simulink model "bh_rolling_wheel_sim_simscape"  (R2022b)
settings: Solver=ode15s  StartTime=0.0  StopTime=15  RelTol=1e-6  AbsTol=1e-5  EnableMultiTasking=on
values from neighbouring files (symbols this model uses):
  X = OBJ.X_g_birth_wheel    [bh_rolling_wheel_toy_CLS.m]
  Y = OBJ.Y_g_birth_wheel    [bh_rolling_wheel_toy_CLS.m]
  Z = OBJ.Z_g_birth_wheel    [bh_rolling_wheel_toy_CLS.m]
undefined symbols (not defined in the file or in its folder): params_T
libraries: sm_lib x9, nesl_utility x7
settings Model: Creator=bhorton  LastModifiedBy=bhorton
settings SolverCC: ZeroCrossAlgorithm=Adaptive  AlgebraicLoopSolver=TrustRegion
settings DataIOCC: LimitDataPoints=on  MaxDataPoints=10000
settings OptimizationCC: LifeSpan=inf
settings DebuggingCC: UnconnectedInputMsg=warning  UnconnectedOutputMsg=warning  UnconnectedLineMsg=warning  AllowSymbolicDim=off  SFUnexpectedBacktrackingDiag=warning  SFNoUnconditionalDefaultTransitionDiag=warning  SFExecutionAtInitializationDiag=none  SFMachineParentedDataDiag=warning  ArithmeticOperatorsInVariantConditions=warning
settings ModelReferenceCC: EnableRefExpFcnMdlSchedulingChecks=on
settings SFSimCC: SimUseLocalCustomCode=off  CustomCodeUndefinedFunction=UseInterfaceOnly
settings RTWCC: RTWUseLocalCustomCode=off  DLArmComputeVersion=19.05
settings CodeAppCC: StateflowObjectComments=on
settings GRTTargetCC: TargetLangStandard=C89/C90 (ANSI)
settings ConfigComp: CovMetricSettings=dw  CovSaveCumulativeToWorkspaceVar=on  CovSaveSingleToWorkspaceVar=on  CovExternalEMLEnable=off  CovSFcnEnable=off
settings SimscapeCC: SimscapeLogType=all  SimscapeLogSimulationStatistics=on  SimscapeLogDataHistory=10000
settings ExplorerConfigSet: InternalSimMechanicsExplorerSettings="<ExplorerConfiguration><canonicalview>default</canonicalview><AnimationSetting><BasePlaybackSpeed>1.0</BasePlaybackSpeed><PlaybackSpeedFactor>1.0</PlaybackSpeedFactor></AnimationSetting><TilePanel><TileInfo><Tiles Columns=\"2\" Count=\"3\" Rows=\"2\"><Column Weight=\"0.5\"/><Column Weight=\"0.5\"/><Row Weight=\"0.4994\"/><Row Weight=\"0.5006\"/><Tile Height=\"1\" Width=\"2\" X=\"0\" Y=\"0\"/><Tile Height=\"1\" Width=\"1\" X=\"0\" Y=\"1\"/><Tile Height=\"1\" Width=\"1\" X=\"1\" Y=\"1\"/></Tiles></TileInfo><SceneInfo><SceneViewer><BGColor><R>0.60000002384185791</R><G>0.60000002384185791</G><B>0.60000002384185791</B></BGColor><Camera><DoPerspective>off</DoPerspective><Position><X>-1.55053169967245363</X><Y>-3.57091267042787441</Y><Z>1.79762407921706791</Z></Position><Center><X>0.0298580117792944799</X><Y>0.315652701739378039</Y><Z>0.371428906966243755</Z></Center><Up><X>0.188235579796397878</X><Y>0.269970042606700877</Y><Z>0.944289967432488608</Z></Up><ViewLimDist>1</ViewLimDist><YLim>2.36177470231108044</YLim><XLim>4.53695320917997602</XLim></Camera></SceneViewer><SceneViewer><BGColor><R>0.60000002384185791</R><G>0.60000002384185791</G><B>0.60000002384185791</B></BGColor><Camera><DoPerspective>off</DoPerspective><Position><X>7.9175910466799948e-08</X><Y>4.21699887787063687e-08</Y><Z>4.27096389083537709</Z></Position><Center><X>7.9175910466799948e-08</X><Y>4.21699887787063687e-08</Y><Z>0.410300941791907015</Z></Center><Up><X>0</X><Y>1</Y><Z>-0</Z></Up><ViewLimDist>1</ViewLimDist><YLim>3.25881235154394311</YLim><XLim>3.08999999999999986</XLim></Camera></SceneViewer><SceneViewer><BGColor><R>0.60000002384185791</R><G>0.60000002384185791</G><B>0.60000002384185791</B></BGColor><Camera><DoPerspective>off</DoPerspective><Position><X>2.4535844008356591</X><Y>-2.45358462381710618</Y><Z>2.45358456126027713</Z></Position><Center><X>-1.19276180646206974e-07</X><Y>-1.03705266674473913e-07</Y><Z>4.11484375746999591e-08</Z></Center><Up><X>-0.408248290463863073</X><Y>0.408248290463863073</Y><Z>0.816496580927726145</Z></Up><ViewLimDist>1</ViewLimDist><YLim>4.60865641641503565</YLim><XLim>4.36991971015930147</XLim></Camera></SceneViewer></SceneInfo></TilePanel><MechEditorPanel><Cameras/><GfxPanelCameraMap/><VideoCreator><PlaybackSpeedRatio>1.0</PlaybackSpeedRatio><FrameRate>30</FrameRate><VideoFormat>Motion JPEG AVI</VideoFormat><FrameSize>auto</FrameSize></VideoCreator></MechEditorPanel></ExplorerConfiguration>"

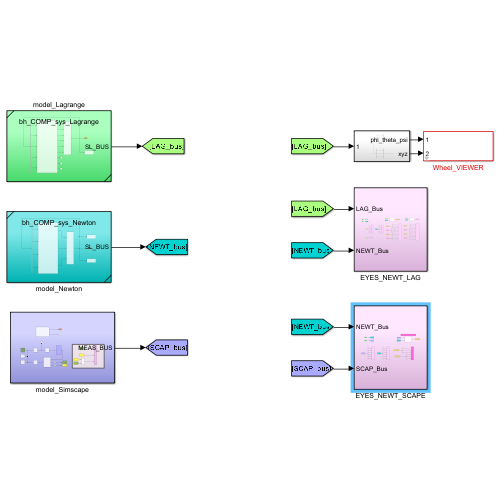
[thumbnail: Simulink's stored preview of the top-level diagram]
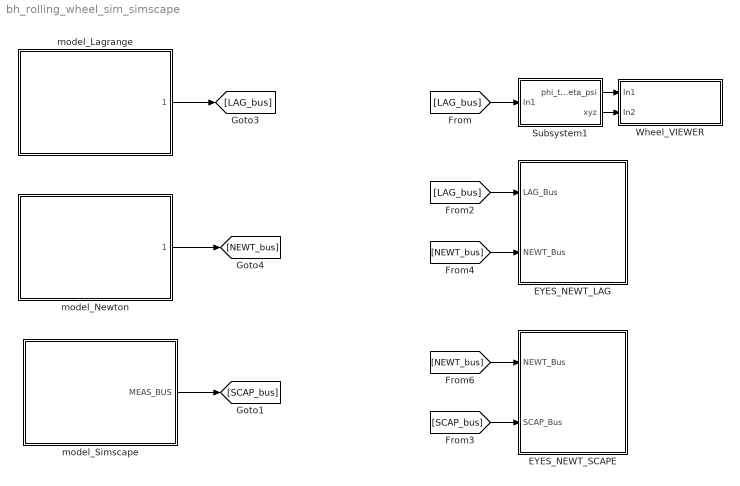
== system bh_rolling_wheel_sim_simscape ==
  EYES_NEWT_LAG : Subsystem
  EYES_NEWT_SCAPE : Subsystem
  Subsystem1 : Subsystem
  Wheel_VIEWER : Subsystem  mask{Ts=0.01, R=params_T.r, the_XLIM=[-1,1]*3, the_YLIM=[-1,1]*3, yn_create_gif=off}
      mask prompts: Ts "Sample Time"; R "Wheel radius (m)"; the_XLIM "X axis display limita"; the_YLIM "Y axis display limita"; yn_create_gif "Create a Gif animation"
      mask init:
      | tf_create_gif = false;
      | 
      | if(1 == yn_create_gif)
      |     tf_create_gif = true;
      | end
  model_Lagrange : Subsystem  ReferencedSubsystem=bh_COMP_sys_Lagrange
  model_Newton : Subsystem  ReferencedSubsystem=bh_COMP_sys_Newton
  model_Simscape : Subsystem
  wires:
  model_Lagrange/1 -> [LAG_bus]
  [LAG_bus] -> EYES_NEWT_LAG/1(LAG_Bus)
  model_Newton/1 -> [NEWT_bus]
  [NEWT_bus] -> EYES_NEWT_LAG/2(NEWT_Bus)
  [LAG_bus] -> Subsystem1/1(In1)
  Subsystem1/1(phi_theta_psi) -> Wheel_VIEWER/1(In1)
  Subsystem1/2(xyz) -> Wheel_VIEWER/2(In2)
  model_Simscape/1(MEAS_BUS) -> [SCAP_bus]
  [NEWT_bus] -> EYES_NEWT_SCAPE/1(NEWT_Bus)
  [SCAP_bus] -> EYES_NEWT_SCAPE/2(SCAP_Bus)

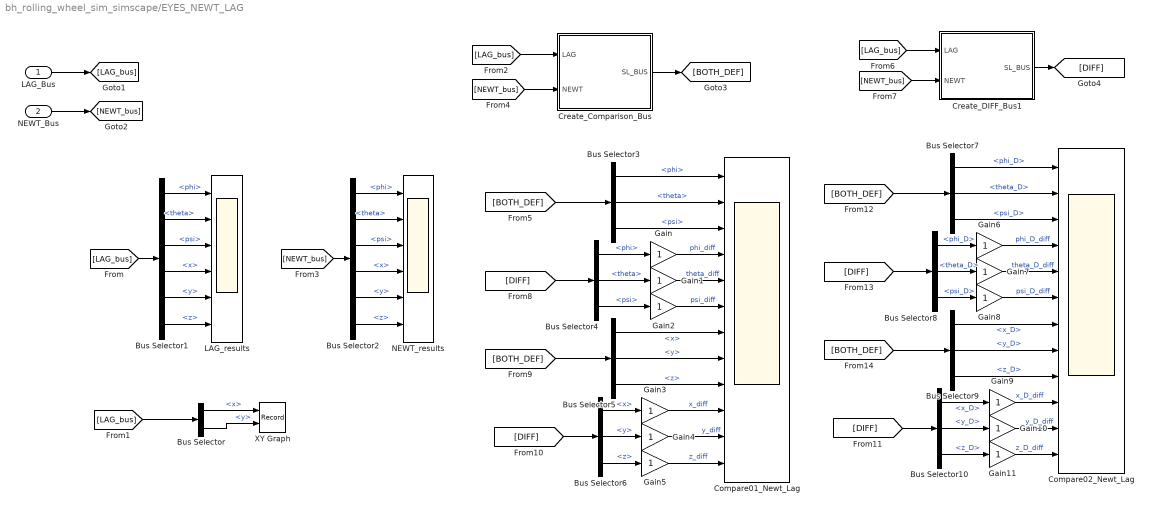
== system bh_rolling_wheel_sim_simscape/EYES_NEWT_LAG ==
  LAG_Bus : Inport
  NEWT_Bus : Inport  Port=2
  Bus Selector : BusSelector  OutputSignals=x,y
  Bus Selector1 : BusSelector  OutputSignals=phi,theta,psi,x,y,z
  Bus Selector10 : BusSelector  OutputSignals=x_D,y_D,z_D
  Bus Selector2 : BusSelector  OutputSignals=phi,theta,psi,x,y,z
  Bus Selector3 : BusSelector  OutputSignals=phi,theta,psi
  Bus Selector4 : BusSelector  OutputSignals=phi,theta,psi
  Bus Selector5 : BusSelector  OutputSignals=x,y,z
  Bus Selector6 : BusSelector  OutputSignals=x,y,z
  Bus Selector7 : BusSelector  OutputSignals=phi_D,theta_D,psi_D
  Bus Selector8 : BusSelector  OutputSignals=phi_D,theta_D,psi_D
  Bus Selector9 : BusSelector  OutputSignals=x_D,y_D,z_D
  Compare01_Newt_Lag : Scope  NumInputPorts=12
  Compare02_Newt_Lag : Scope  NumInputPorts=12
  Create_Comparison_Bus : Subsystem
  Create_DIFF_Bus1 : Subsystem
  Gain{,1..11} (12 alike) : Gain
  LAG_results : Scope  NumInputPorts=6
  NEWT_results : Scope  NumInputPorts=6
  XY Graph : Record  FileSettingsInternal="{\"entries\":[{\"content\":{\"excelSettings\":{\"content\":{},\"type\":\"Streamout.ExcelSettings\"}},\"type\":\"Streamout.FileSettingStorage\",\"uuid\":\"1ddb2a88-b2ea-40b8-bd98-e1e8a9863809\"}],\"packageUris\":[\"http://schema.mathworks.com/mf0/streamout_blocks/R2020a\"],\"version\":\"1.0\"}"  Layout=[1 1]  SignalsInternal="{\"entries\":[{\"content\":{\"signals\":[{\"content\":{\"blockPath\":[\"bh_rolling_wheel_sim_simscape/EYES_NEWT_LAG/XY Graph\"],\"channel\":[],\"dimensions\":[1],\"domain\":\"bh_rolling_wheel_sim_simscape/EYES_NEWT_LAG/XY Graph\",\"lineColor\":\"#edb120\",\"plots\":[],\"port\":1,\"sid\":[],\"signalID\":846,\"signalName\":\"<x>\"},\"type\":\"RecordBlkView.Signal\",\"uuid\":\"96332ea5-5fdc-4ca9-b00e-a419accddd88\"},{\"content\":{\"blockPath\":[\"bh_rolling_wheel_sim_simscape/EYES_NEWT_LAG/XY Graph\"],\"channel\":[],\"dimensions\":[1],\"domain\":\"bh_rolling_wheel_sim_simscape/EYES_NEWT_LAG/XY Graph\",\"lineColor\":\"#7e2f8e\",\"plots\":[],\"port\":2,\"sid\":[],\"signalID\":849,\"signalName\":\"<y>\"},\"type\":\"RecordBlkView.Signal\",\"uuid\":\"f7c696c0-69e3-4450-bb2d-fd5414803194\"}]},\"type\":\"RecordBlkView.InputSignals\",\"uuid\":\"ee3b015f-a261-4ccc-b071-21c734062a7a\"}],\"packageUris\":[\"http://schema.mathworks.com/mf0/streamout_blocks/R2020a\"],\"version\":\"1.0\"}"  VisualizationBindings="{\"xyplotplugin\":{\"info\":[{\"series\":[],\"subplotID\":1}]}}"  CompatibilityTag=XY  st=-1
  wires:
  LAG_Bus/1 -> [LAG_bus]
  [LAG_bus] -> Bus Selector1/1
  Bus Selector1/1 -> LAG_results/1  "<phi>"
  Bus Selector1/2 -> LAG_results/2  "<theta>"
  Bus Selector1/3 -> LAG_results/3  "<psi>"
  Bus Selector1/4 -> LAG_results/4  "<x>"
  Bus Selector1/5 -> LAG_results/5  "<y>"
  Bus Selector1/6 -> LAG_results/6  "<z>"
  [LAG_bus] -> Bus Selector/1
  Bus Selector/1 -> XY Graph/1  "<x>"
  Bus Selector/2 -> XY Graph/2  "<y>"
  NEWT_Bus/1 -> [NEWT_bus]
  Bus Selector2/5 -> NEWT_results/5  "<y>"
  Bus Selector2/4 -> NEWT_results/4  "<x>"
  Bus Selector2/2 -> NEWT_results/2  "<theta>"
  Bus Selector2/1 -> NEWT_results/1  "<phi>"
  Bus Selector2/6 -> NEWT_results/6  "<z>"
  [NEWT_bus] -> Bus Selector2/1
  Bus Selector2/3 -> NEWT_results/3  "<psi>"
  Create_Comparison_Bus/1(SL_BUS) -> [BOTH_DEF]
  [NEWT_bus] -> Create_Comparison_Bus/2(NEWT)
  [LAG_bus] -> Create_Comparison_Bus/1(LAG)
  [NEWT_bus] -> Create_DIFF_Bus1/2(NEWT)
  [LAG_bus] -> Create_DIFF_Bus1/1(LAG)
  Create_DIFF_Bus1/1(SL_BUS) -> [DIFF]
  [BOTH_DEF] -> Bus Selector3/1
  Bus Selector3/1 -> Compare01_Newt_Lag/1  "<phi>"
  Bus Selector3/2 -> Compare01_Newt_Lag/2  "<theta>"
  Bus Selector3/3 -> Compare01_Newt_Lag/3  "<psi>"
  Bus Selector4/1 -> Gain/1  "<phi>"
  Bus Selector4/2 -> Gain1/1  "<theta>"
  Bus Selector4/3 -> Gain2/1  "<psi>"
  [DIFF] -> Bus Selector4/1
  [BOTH_DEF] -> Bus Selector5/1
  Bus Selector5/1 -> Compare01_Newt_Lag/7  "<x>"
  Bus Selector5/2 -> Compare01_Newt_Lag/8  "<y>"
  Bus Selector5/3 -> Compare01_Newt_Lag/9  "<z>"
  Bus Selector6/2 -> Gain4/1  "<y>"
  [DIFF] -> Bus Selector6/1
  Bus Selector6/1 -> Gain3/1  "<x>"
  Bus Selector6/3 -> Gain5/1  "<z>"
  Bus Selector9/1 -> Compare02_Newt_Lag/7  "<x_D>"
  [BOTH_DEF] -> Bus Selector9/1
  Bus Selector9/3 -> Compare02_Newt_Lag/9  "<z_D>"
  Bus Selector9/2 -> Compare02_Newt_Lag/8  "<y_D>"
  Bus Selector7/1 -> Compare02_Newt_Lag/1  "<phi_D>"
  Bus Selector7/2 -> Compare02_Newt_Lag/2  "<theta_D>"
  Bus Selector7/3 -> Compare02_Newt_Lag/3  "<psi_D>"
  [DIFF] -> Bus Selector8/1
  [DIFF] -> Bus Selector10/1
  [BOTH_DEF] -> Bus Selector7/1
  Gain2/1 -> Compare01_Newt_Lag/6  "psi_diff"
  Gain/1 -> Compare01_Newt_Lag/4  "phi_diff"
  Gain1/1 -> Compare01_Newt_Lag/5  "theta_diff"
  Gain3/1 -> Compare01_Newt_Lag/10  "x_diff"
  Gain4/1 -> Compare01_Newt_Lag/11  "y_diff"
  Gain5/1 -> Compare01_Newt_Lag/12  "z_diff"
  Bus Selector8/1 -> Gain6/1  "<phi_D>"
  Bus Selector8/2 -> Gain7/1  "<theta_D>"
  Bus Selector8/3 -> Gain8/1  "<psi_D>"
  Bus Selector10/1 -> Gain9/1  "<x_D>"
  Bus Selector10/2 -> Gain10/1  "<y_D>"
  Bus Selector10/3 -> Gain11/1  "<z_D>"
  Gain6/1 -> Compare02_Newt_Lag/4  "phi_D_diff"
  Gain7/1 -> Compare02_Newt_Lag/5  "theta_D_diff"
  Gain8/1 -> Compare02_Newt_Lag/6  "psi_D_diff"
  Gain9/1 -> Compare02_Newt_Lag/10  "x_D_diff"
  Gain10/1 -> Compare02_Newt_Lag/11  "y_D_diff"
  Gain11/1 -> Compare02_Newt_Lag/12  "z_D_diff"

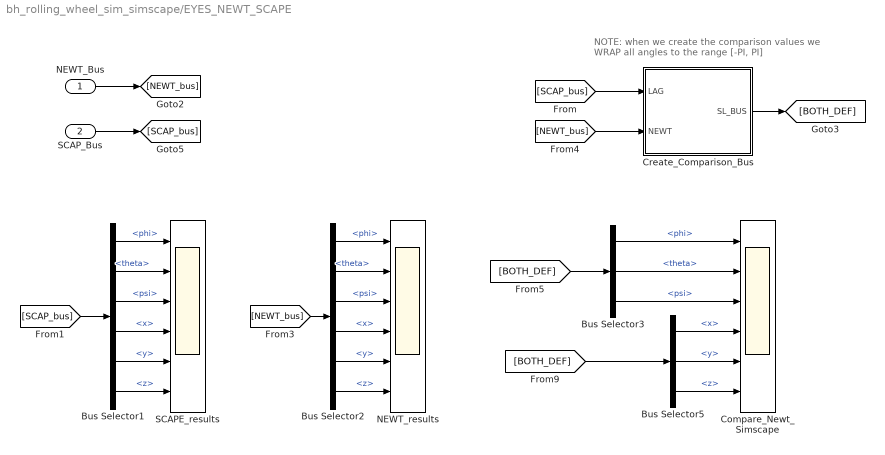
== system bh_rolling_wheel_sim_simscape/EYES_NEWT_SCAPE ==
  note: NOTE:  when we create the comparison values
      | we WRAP all angles to the range [-PI, PI]
  NEWT_Bus : Inport
  SCAP_Bus : Inport  Port=2
  Bus Selector1 : BusSelector  OutputSignals=phi,theta,psi,x,y,z
  Bus Selector2 : BusSelector  OutputSignals=phi,theta,psi,x,y,z
  Bus Selector3 : BusSelector  OutputSignals=phi,theta,psi
  Bus Selector5 : BusSelector  OutputSignals=x,y,z
  Compare_Newt_Simscape : Scope  NumInputPorts=6
  Create_Comparison_Bus : Subsystem
  NEWT_results : Scope  NumInputPorts=6
  SCAPE_results : Scope  NumInputPorts=6
  wires:
  [SCAP_bus] -> Bus Selector1/1
  Bus Selector1/1 -> SCAPE_results/1  "<phi>"
  Bus Selector1/2 -> SCAPE_results/2  "<theta>"
  Bus Selector1/3 -> SCAPE_results/3  "<psi>"
  Bus Selector1/4 -> SCAPE_results/4  "<x>"
  Bus Selector1/5 -> SCAPE_results/5  "<y>"
  Bus Selector1/6 -> SCAPE_results/6  "<z>"
  NEWT_Bus/1 -> [NEWT_bus]
  Bus Selector2/5 -> NEWT_results/5  "<y>"
  Bus Selector2/4 -> NEWT_results/4  "<x>"
  Bus Selector2/2 -> NEWT_results/2  "<theta>"
  Bus Selector2/1 -> NEWT_results/1  "<phi>"
  Bus Selector2/6 -> NEWT_results/6  "<z>"
  [NEWT_bus] -> Bus Selector2/1
  Bus Selector2/3 -> NEWT_results/3  "<psi>"
  Create_Comparison_Bus/1(SL_BUS) -> [BOTH_DEF]
  [NEWT_bus] -> Create_Comparison_Bus/2(NEWT)
  [SCAP_bus] -> Create_Comparison_Bus/1(LAG)
  [BOTH_DEF] -> Bus Selector3/1
  Bus Selector3/1 -> Compare_Newt_Simscape/1  "<phi>"
  Bus Selector3/2 -> Compare_Newt_Simscape/2  "<theta>"
  Bus Selector3/3 -> Compare_Newt_Simscape/3  "<psi>"
  [BOTH_DEF] -> Bus Selector5/1
  Bus Selector5/1 -> Compare_Newt_Simscape/4  "<x>"
  Bus Selector5/2 -> Compare_Newt_Simscape/5  "<y>"
  Bus Selector5/3 -> Compare_Newt_Simscape/6  "<z>"
  SCAP_Bus/1 -> [SCAP_bus]

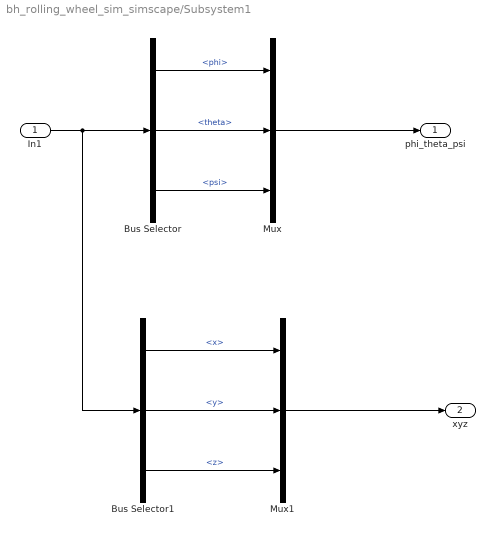
== system bh_rolling_wheel_sim_simscape/Subsystem1 ==
  In1 : Inport
  Bus Selector : BusSelector  OutputSignals=phi,theta,psi
  Bus Selector1 : BusSelector  OutputSignals=x,y,z
  Mux : Mux  Inputs=3
  Mux1 : Mux  Inputs=3
  phi_theta_psi : Outport
  xyz : Outport  Port=2
  wires:
  In1/1 -> Bus Selector1/1, Bus Selector/1
  Bus Selector/1 -> Mux/1  "<phi>"
  Bus Selector/2 -> Mux/2  "<theta>"
  Bus Selector/3 -> Mux/3  "<psi>"
  Bus Selector1/1 -> Mux1/1  "<x>"
  Bus Selector1/2 -> Mux1/2  "<y>"
  Bus Selector1/3 -> Mux1/3  "<z>"
  Mux/1 -> phi_theta_psi/1
  Mux1/1 -> xyz/1

== system bh_rolling_wheel_sim_simscape/Wheel_VIEWER ==
  In1 : Inport
  In2 : Inport  Port=2
  Level-2 MATLAB S-Function : M-S-Function  FunctionName=bh_rolling_wheel_animate_sfun  Parameters=Ts, R, the_XLIM, the_YLIM, tf_create_gif
  wires:
  In1/1 -> Level-2 MATLAB S-Function/1
  In2/1 -> Level-2 MATLAB S-Function/2

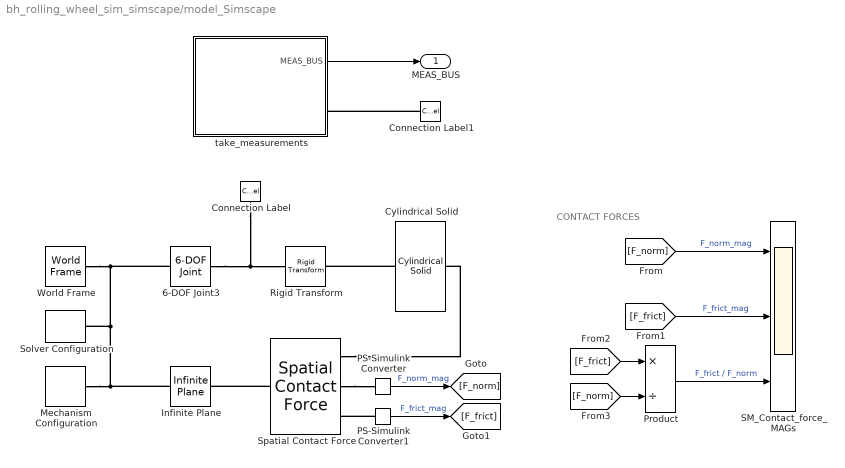
== system bh_rolling_wheel_sim_simscape/model_Simscape ==
  note: CONTACT FORCES
  6-DOF Joint3 : sm_lib/Joints/6-DOF Joint  JointMode=Normal  SenseConstraintForce=off  SenseConstraintForceX=off  SenseConstraintForceY=off  SenseConstraintForceZ=off  SenseConstraintTorque=off  SenseConstraintTorqueX=off  SenseConstraintTorqueY=off  SenseConstraintTorqueZ=off  SenseTotalForce=off  SenseTotalForceX=off  SenseTotalForceY=off  SenseTotalForceZ=off  SenseTotalTorque=off  SenseTotalTorqueX=off  SenseTotalTorqueY=off  SenseTotalTorqueZ=off  CompositeWrenchDir=FollowerOnBase  CompositeWrenchFrame=BaseFrame  PxEquilibriumPosition=0  PxEquilibriumPositionUnits=m  PxSpringStiffness=0  PxSpringStiffnessUnits=N/m  PxDampingCoefficient=0  PxDampingCoefficientUnits=N/(m/s)  PxTorqueActuationMode=NoTorque  PxMotionActuationMode=ComputedMotion  PxSensePosition=off  PxSenseVelocity=off  PxSenseAcceleration=off  PxSenseTorqueForce=off  PxSenseLowerLimitTorqueForce=off  PxSenseUpperLimitTorqueForce=off  PxLowerLimitSpecify=off  PxLowerLimitBound=-1  PxLowerLimitBoundUnits=m  PxLowerLimitStiffness=1e6  PxLowerLimitStiffnessUnits=N/m  PxLowerLimitDamping=1e3  PxLowerLimitDampingUnits=N/(m/s)  PxLowerLimitTransitionRegionWidth=1e-4  PxLowerLimitTransitionRegionWidthUnits=m  PxUpperLimitSpecify=off  PxUpperLimitBound=1  PxUpperLimitBoundUnits=m  PxUpperLimitStiffness=1e6  PxUpperLimitStiffnessUnits=N/m  PxUpperLimitDamping=1e3  PxUpperLimitDampingUnits=N/(m/s)  PxUpperLimitTransitionRegionWidth=1e-4  PxUpperLimitTransitionRegionWidthUnits=m  PxPositionTargetSpecify=on  PxPositionTargetPriority=High  PxPositionTargetValue=IC_T.x  PxPositionTargetValueUnits=m  PxVelocityTargetSpecify=on  PxVelocityTargetPriority=High  PxVelocityTargetValue=IC_T.x_dot  PxVelocityTargetValueUnits=m/s  PyEquilibriumPosition=0  PyEquilibriumPositionUnits=m  PySpringStiffness=0  PySpringStiffnessUnits=N/m  PyDampingCoefficient=0  PyDampingCoefficientUnits=N/(m/s)  PyTorqueActuationMode=NoTorque  PyMotionActuationMode=ComputedMotion  PySensePosition=off  PySenseVelocity=off  PySenseAcceleration=off  PySenseTorqueForce=off  PySenseLowerLimitTorqueForce=off  PySenseUpperLimitTorqueForce=off  PyLowerLimitSpecify=off  PyLowerLimitBound=-1  PyLowerLimitBoundUnits=m  PyLowerLimitStiffness=1e6  PyLowerLimitStiffnessUnits=N/m  PyLowerLimitDamping=1e3  PyLowerLimitDampingUnits=N/(m/s)  PyLowerLimitTransitionRegionWidth=1e-4  PyLowerLimitTransitionRegionWidthUnits=m  PyUpperLimitSpecify=off  PyUpperLimitBound=1  PyUpperLimitBoundUnits=m  PyUpperLimitStiffness=1e6  PyUpperLimitStiffnessUnits=N/m  PyUpperLimitDamping=1e3  PyUpperLimitDampingUnits=N/(m/s)  PyUpperLimitTransitionRegionWidth=1e-4  PyUpperLimitTransitionRegionWidthUnits=m  PyPositionTargetSpecify=on  PyPositionTargetPriority=High  PyPositionTargetValue=IC_T.y  PyPositionTargetValueUnits=m  PyVelocityTargetSpecify=on  PyVelocityTargetPriority=High  PyVelocityTargetValue=IC_T.y_dot  PyVelocityTargetValueUnits=m/s  PzEquilibriumPosition=0  PzEquilibriumPositionUnits=m  PzSpringStiffness=0  PzSpringStiffnessUnits=N/m  PzDampingCoefficient=0  PzDampingCoefficientUnits=N/(m/s)  PzTorqueActuationMode=NoTorque  PzMotionActuationMode=ComputedMotion  PzSensePosition=off  PzSenseVelocity=off  PzSenseAcceleration=off  PzSenseTorqueForce=off  PzSenseLowerLimitTorqueForce=off  PzSenseUpperLimitTorqueForce=off  PzLowerLimitSpecify=off  PzLowerLimitBound=-1  PzLowerLimitBoundUnits=m  PzLowerLimitStiffness=1e6  PzLowerLimitStiffnessUnits=N/m  PzLowerLimitDamping=1e3  PzLowerLimitDampingUnits=N/(m/s)  PzLowerLimitTransitionRegionWidth=1e-4  PzLowerLimitTransitionRegionWidthUnits=m  PzUpperLimitSpecify=off  PzUpperLimitBound=1  PzUpperLimitBoundUnits=m  PzUpperLimitStiffness=1e6  PzUpperLimitStiffnessUnits=N/m  PzUpperLimitDamping=1e3  PzUpperLimitDampingUnits=N/(m/s)  PzUpperLimitTransitionRegionWidth=1e-4  PzUpperLimitTransitionRegionWidthUnits=m  PzPositionTargetSpecify=on  PzPositionTargetPriority=High  PzPositionTargetValue=IC_T.z  PzPositionTargetValueUnits=m  PzVelocityTargetSpecify=on  PzVelocityTargetPriority=High  PzVelocityTargetValue=IC_T.z_dot  PzVelocityTargetValueUnits=m/s  SphEqPosRotationMethod=None  SphEqPosRotationAngleUnits=deg  SphEqPosRotationStandardAxis=+Z  SphEqPosRotationAngle=0.0  SphEqPosRotationArbitraryAxis=[0 0 1]  SphEqPosFollAlignAxisA=+X  SphEqPosBaseAlignAxisA=+Y  SphEqPosFollAlignAxisB=+Y  SphEqPosBaseAlignAxisB=+Z  SphEqPosRotationSequenceAxes=FollowerAxes  SphEqPosRotationSequence=XYX  SphEqPosRotationSequenceAngles=[0 0 0]  SphEqPosRotationSequenceAnglesUnits=deg  SphEqPosRotationMatrix=[1 0 0; 0 1 0; 0 0 1]  SphEqPosQuaternion=[1 0 0 0]  SphSpringStiffness=0  SphSpringStiffnessUnits=N*m/deg  SphDampingCoefficient=0  SphDampingCoefficientUnits=N*m/(deg/s)  SphActuateTorqueX=off  SphActuateTorqueY=off  SphActuateTorqueZ=off  SphActuateTorque=off  SphTorqueActuationMode=NoTorque  SphMotionActuationMode=ComputedMotion  SphActuationFrame=BaseFrame  SphSensePosition=off  SphSenseVelocityX=off  SphSenseVelocityY=off  SphSenseVelocityZ=off  SphSenseVelocity=off  SphSenseAccelerationX=off  SphSenseAccelerationY=off  SphSenseAccelerationZ=off  SphSenseAcceleration=off  SphSenseTorqueX=off  SphSenseTorqueY=off  SphSenseTorqueZ=off  SphSenseTorqueForce=off  SphSenseLowerLimitTorqueMag=off  SphSenseUpperLimitTorqueMag=off  SphSensingFrame=BaseFrame  SphLowerLimitSpecify=off  SphLowerLimitBound=15  SphLowerLimitBoundUnits=deg  SphLowerLimitStiffness=1e4  SphLowerLimitStiffnessUnits=N*m/deg  SphLowerLimitDamping=10  SphLowerLimitDampingUnits=N*m/(deg/s)  SphLowerLimitTransitionRegionWidth=0.1  SphLowerLimitTransitionRegionWidthUnits=deg  SphUpperLimitSpecify=off  SphUpperLimitBound=45  SphUpperLimitBoundUnits=deg  SphUpperLimitStiffness=1e4  SphUpperLimitStiffnessUnits=N*m/deg  SphUpperLimitDamping=10  SphUpperLimitDampingUnits=N*m/(deg/s)  SphUpperLimitTransitionRegionWidth=0.1  SphUpperLimitTransitionRegionWidthUnits=deg  SphPositionTargetRotationMethod=RotationSequence  SphPositionTargetRotationAngleUnits=deg  SphPositionTargetRotationStandardAxis=+Z  SphPositionTargetRotationAngle=0.0  SphPositionTargetRotationArbitraryAxis=[0 0 1]  SphPositionTargetFollAlignAxisA=+X  SphPositionTargetBaseAlignAxisA=+Y  SphPositionTargetFollAlignAxisB=+Y  SphPositionTargetBaseAlignAxisB=+Z  SphPositionTargetRotationSequenceAxes=FollowerAxes  SphPositionTargetRotationSequence=ZYX  SphPositionTargetRotationSequenceAngles=IC_T.rot_ang_ZYX  SphPositionTargetRotationSequenceAnglesUnits=rad  SphPositionTargetRotationMatrix=[1 0 0; 0 1 0; 0 0 1]  SphPositionTargetQuaternion=[1 0 0 0]  SphPositionTargetSpecify=on  SphPositionTargetPriority=High  SphVelocityTargetValue=IC_T.rot_vel_ZYX  SphVelocityTargetValueUnits=rad/s  SphVelocityTargetSpecify=on  SphVelocityTargetPriority=High  SphVelocityTargetInFollowerFrame=on
  Connection Label : ConnectionLabel  Label=CoM
  Connection Label1 : ConnectionLabel  Label=CoM
  Cylindrical Solid : sm_lib/Body Elements/Cylindrical Solid  GraphicAmbientColor=[0.15 0.15 0.15 1.0]  BasedOnType=Mass  CenterOfMass=[0 0 0]  CenterOfMassUnits=m  GraphicDiffuseColor=[0.6 0.6 1.0]  CylinderLength=params_T.r/100  CylinderLengthUnits=m  CylinderRadius=params_T.r  CylinderRadiusUnits=m  Density=1000  DensityUnits=kg/m^3  DoExposeReferenceFrame=on  GraphicEmissiveColor=[0.0 0.0 0.0 1.0]  ExportEntireGeometry=on  SerializedFrames=<Frames/>  MarkerShape=Sphere  MarkerSize=10  GraphicType=FromGeometry  InertiaType=Custom  Mass=params_T.m  MassUnits=kg  MomentsOfInertia=params.I_mome_for_simscape  MomentsOfInertiaUnits=kg*m^2  GraphicOpacity=1.0  ProductsOfInertia=params.I_prod_for_simscape  ProductsOfInertiaUnits=kg*m^2  GraphicShininess=75  GraphicSpecularColor=[0.5 0.5 0.5 1.0]  GraphicVisPropType=SimpleVisualProperties
  Infinite Plane : sm_lib/Curves and Surfaces/Infinite Plane  GraphicType=Rectangle  GraphicPlaneWidth=6  GraphicPlaneWidthUnits=m  GraphicPlaneHeight=6  GraphicPlaneHeightUnits=m  GraphicVisPropType=SimpleVisualProperties  GraphicDiffuseColor=[0.5 0.5 0.5]  GraphicOpacity=0.25  GraphicSpecularColor=[0.5 0.5 0.5 1.0]  GraphicAmbientColor=[0.15 0.15 0.15 1.0]  GraphicEmissiveColor=[0.0 0.0 0.0 1.0]  GraphicShininess=75
  Mechanism Configuration : sm_lib/Utilities/Mechanism Configuration  UniformGravity=Constant  GravityVector=[0 0 -9.80665]  GravityUnits=m/s^2  LinearizationDelta=0.001  JointModeTransitionNonlinearIterations=2
  PS-Simulink Converter : nesl_utility/PS-Simulink Converter  PhysicalDomain=network_engine_domain  SubClassName=ps_output  LeftPortType=input  RightPortType=output  PseudoPeriodic=off  Frequencies=[]  VectorFormat=1-D array  Unit=N  AffineConversion=off
  PS-Simulink Converter1 : nesl_utility/PS-Simulink Converter  PhysicalDomain=network_engine_domain  SubClassName=ps_output  LeftPortType=input  RightPortType=output  PseudoPeriodic=off  Frequencies=[]  VectorFormat=1-D array  Unit=N  AffineConversion=off
  Product : Product  Inputs=*/
  Rigid Transform : sm_lib/Frames and Transforms/Rigid Transform  TranslationMethod=None  TranslationStandardOffset=0  TranslationLengthUnit=m  TranslationStandardAxis=+Z  TranslationCartesianOffset=[0 0 0]  TranslationROffset=0  TranslationROffsetUnits=m  TranslationZOffset=0  TranslationZOffsetUnits=m  TranslationThetaOffset=0  TranslationThetaOffsetUnits=deg  RotationMethod=AlignedAxes  RotationAngleUnits=deg  RotationStandardAxis=+Z  RotationAngle=0.0  RotationArbitraryAxis=[0 0 1]  FollAlignAxisA=+Y  BaseAlignAxisA=+Z  FollAlignAxisB=+X  BaseAlignAxisB=+Y  RotationSequenceAxes=FollowerAxes  RotationSequence=XYX  RotationSequenceAngles=[0 0 0]  RotationSequenceAnglesUnits=deg  RotationMatrix=[1 0 0; 0 1 0; 0 0 1]  Quaternion=[1 0 0 0]
  SM_Contact_force_MAGs : Scope  NumInputPorts=3
  Solver Configuration : nesl_utility/Solver Configuration  PhysicalDomain=network_engine_domain  SubClassName=solver  LeftPortType=input  RightPortType=generic  Tones=[]  Harmonics=[]  SimulateNoise=off  Profile=off  UseLocalSampling=off  EnableSwitchedLinearOptims=on  FrequencyDomain=off  UseCCode=off  RelTol=0.001  AbsTol=1e-06  MinStep=1e-09  ToWorkspace=off  RevertToSquareIcSolve=off  NumHomotopyIterations=100  PhasorMode=off  PhasorModeNumHarmonics=1  ConsistencySolver=NEWTON_FTOL  IndexReductionMethod=DerivativeReplacement  DoDC=off  ResidualTolerance=1e-09  ConsistencyTolSource=GLOBAL  ConsistencyAbsTol=0.001  ConsistencyRelTol=0.001  ConsistencyTolFactor=0.001  UseLocalSolver=off  LocalSolverChoice=NE_BACKWARD_EULER_ADVANCER  ResolveIndetEquations=on  FunctionEvalNumThread=1  LocalSolverSampleTime=0.001  DoFixedCost=off  MaxNonlinIter=3  MaxModeIter=2  ComputeImpulses=off  ImpulseIterations=2  LinearAlgebra=Sparse  LinearAlgebraNumThread=0  EquationFormulation=NE_TIME_EF  DelaysMemoryBudget=1024  AutomaticFiltering=on  FilteringTimeConstant=0.001  PartitionStorageMethod=AS_NEEDED  PartitionMemoryBudget=1024  PartitionMethod=FAST
  Spatial Contact Force : sm_lib/Forces and Torques/Spatial Contact Force  SenseContactBaseRotation=off  SenseContactBaseTranslation=off  CoefficientOfDynamicFriction=contact.Ff_codyn  CoefficientOfStaticFriction=contact.Ff_costat  NormalDamping=contact.Nf_damp  NormalDampingUnits=N/(m/s)  SenseContactSignal=off  NormalStiffness=contact.Nf_stiff  NormalStiffnessUnits=N/m  FrictionalCriticalVelocity=contact.Ff_critvel  FrictionalCriticalVelocityUnits=m/s  ZeroCrossDetectContactStartAndEnd=off  SenseContactFollowerRotation=off  SenseContactFollowerTranslation=off  FrictionType=SmoothStickSlip  SenseFrictionalForceMagnitude=on  SenseNormalForceMagnitude=on  NormalForceType=SmoothSpringDamper  SenseNormalVelocity=off  SenseSeparationDistance=off  SenseTangentialVelocity=off  NormalTransitionRegionWidth=contact.Nf_trwidth  NormalTransitionRegionWidthUnits=m
  World Frame : sm_lib/Frames and Transforms/World Frame
  take_measurements : Subsystem
  MEAS_BUS : Outport
  wires:
  take_measurements/1(MEAS_BUS) -> MEAS_BUS/1
  PS-Simulink Converter/1 -> [F_norm]  "F_norm_mag"
  PS-Simulink Converter1/1 -> [F_frict]  "F_frict_mag"
  Product/1 -> SM_Contact_force_MAGs/3  "F_frict / F_norm"
  [F_frict] -> SM_Contact_force_MAGs/2  "F_frict_mag"
  [F_norm] -> SM_Contact_force_MAGs/1  "F_norm_mag"
  [F_norm] -> Product/2
  [F_frict] -> Product/1
  connections:
  Mechanism Configuration/RConn1 -- Infinite Plane/LConn1 -- World Frame/RConn1 -- 6-DOF Joint3/LConn1 -- Solver Configuration/RConn1
  6-DOF Joint3/RConn1 -- Connection Label/LConn1 -- Rigid Transform/LConn1
  Cylindrical Solid/RConn1 -- Rigid Transform/RConn1
  Spatial Contact Force/LConn1 -- Infinite Plane/RConn1
  Spatial Contact Force/RConn1 -- Cylindrical Solid/LConn1
  Connection Label1/LConn1 -- take_measurements/RConn1
  Spatial Contact Force/RConn2 -- PS-Simulink Converter/LConn1
  PS-Simulink Converter1/LConn1 -- Spatial Contact Force/RConn3

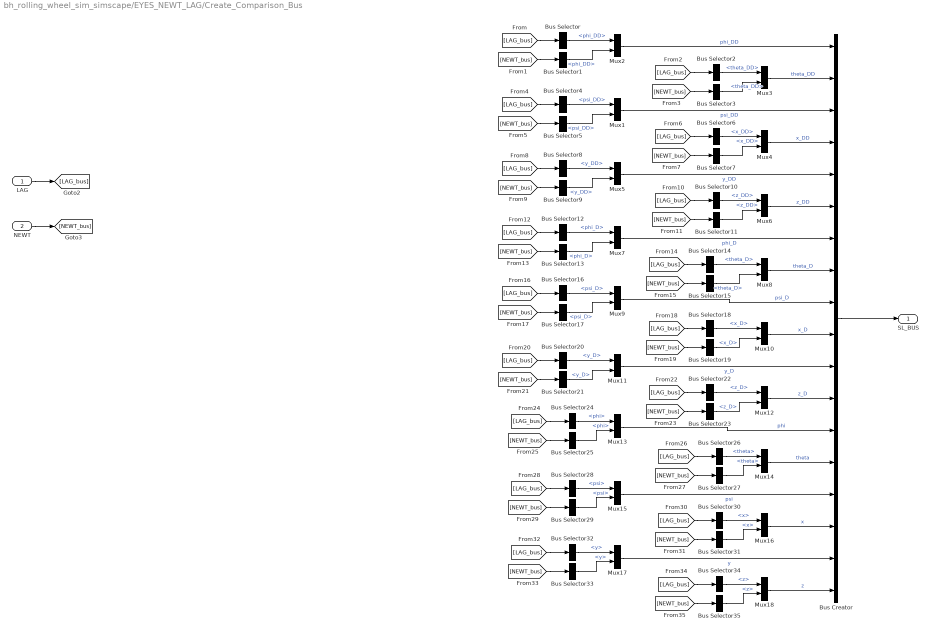
== system bh_rolling_wheel_sim_simscape/EYES_NEWT_LAG/Create_Comparison_Bus ==
  LAG : Inport
  NEWT : Inport  Port=2
  Bus Creator : BusCreator  Inputs=18
  Bus Selector : BusSelector  OutputSignals=phi_DD
  Bus Selector1 : BusSelector  OutputSignals=phi_DD
  Bus Selector10 : BusSelector  OutputSignals=z_DD
  Bus Selector11 : BusSelector  OutputSignals=z_DD
  Bus Selector12 : BusSelector  OutputSignals=phi_D
  Bus Selector13 : BusSelector  OutputSignals=phi_D
  Bus Selector14 : BusSelector  OutputSignals=theta_D
  Bus Selector15 : BusSelector  OutputSignals=theta_D
  Bus Selector16 : BusSelector  OutputSignals=psi_D
  Bus Selector17 : BusSelector  OutputSignals=psi_D
  Bus Selector18 : BusSelector  OutputSignals=x_D
  Bus Selector19 : BusSelector  OutputSignals=x_D
  Bus Selector2 : BusSelector  OutputSignals=theta_DD
  Bus Selector20 : BusSelector  OutputSignals=y_D
  Bus Selector21 : BusSelector  OutputSignals=y_D
  Bus Selector22 : BusSelector  OutputSignals=z_D
  Bus Selector23 : BusSelector  OutputSignals=z_D
  Bus Selector24 : BusSelector  OutputSignals=phi
  Bus Selector25 : BusSelector  OutputSignals=phi
  Bus Selector26 : BusSelector  OutputSignals=theta
  Bus Selector27 : BusSelector  OutputSignals=theta
  Bus Selector28 : BusSelector  OutputSignals=psi
  Bus Selector29 : BusSelector  OutputSignals=psi
  Bus Selector3 : BusSelector  OutputSignals=theta_DD
  Bus Selector30 : BusSelector  OutputSignals=x
  Bus Selector31 : BusSelector  OutputSignals=x
  Bus Selector32 : BusSelector  OutputSignals=y
  Bus Selector33 : BusSelector  OutputSignals=y
  Bus Selector34 : BusSelector  OutputSignals=z
  Bus Selector35 : BusSelector  OutputSignals=z
  Bus Selector4 : BusSelector  OutputSignals=psi_DD
  Bus Selector5 : BusSelector  OutputSignals=psi_DD
  Bus Selector6 : BusSelector  OutputSignals=x_DD
  Bus Selector7 : BusSelector  OutputSignals=x_DD
  Bus Selector8 : BusSelector  OutputSignals=y_DD
  Bus Selector9 : BusSelector  OutputSignals=y_DD
  Mux{1..18} (18 alike) : Mux  Inputs=2
  SL_BUS : Outport
  wires:
  NEWT/1 -> [NEWT_bus]
  LAG/1 -> [LAG_bus]
  [LAG_bus] -> Bus Selector/1
  [NEWT_bus] -> Bus Selector1/1
  Bus Selector/1 -> Mux2/1  "<phi_DD>"
  Bus Selector1/1 -> Mux2/2  "<phi_DD>"
  Mux3/1 -> Bus Creator/2  "theta_DD"
  Mux13/1 -> Bus Creator/13  "phi"
  Mux18/1 -> Bus Creator/18  "z"
  Mux16/1 -> Bus Creator/16  "x"
  Mux15/1 -> Bus Creator/15  "psi"
  Mux9/1 -> Bus Creator/9  "psi_D"
  Mux8/1 -> Bus Creator/8  "theta_D"
  Mux12/1 -> Bus Creator/12  "z_D"
  Mux11/1 -> Bus Creator/11  "y_D"
  Mux17/1 -> Bus Creator/17  "y"
  Mux5/1 -> Bus Creator/5  "y_DD"
  Mux14/1 -> Bus Creator/14  "theta"
  Bus Creator/1 -> SL_BUS/1
  Mux7/1 -> Bus Creator/7  "phi_D"
  Mux10/1 -> Bus Creator/10  "x_D"
  Mux6/1 -> Bus Creator/6  "z_DD"
  Mux4/1 -> Bus Creator/4  "x_DD"
  Mux1/1 -> Bus Creator/3  "psi_DD"
  Mux2/1 -> Bus Creator/1  "phi_DD"
  [LAG_bus] -> Bus Selector2/1
  [NEWT_bus] -> Bus Selector3/1
  Bus Selector2/1 -> Mux3/1  "<theta_DD>"
  Bus Selector3/1 -> Mux3/2  "<theta_DD>"
  Bus Selector5/1 -> Mux1/2  "<psi_DD>"
  [LAG_bus] -> Bus Selector4/1
  Bus Selector4/1 -> Mux1/1  "<psi_DD>"
  [NEWT_bus] -> Bus Selector5/1
  Bus Selector6/1 -> Mux4/1  "<x_DD>"
  [NEWT_bus] -> Bus Selector7/1
  [LAG_bus] -> Bus Selector6/1
  Bus Selector7/1 -> Mux4/2  "<x_DD>"
  Bus Selector8/1 -> Mux5/1  "<y_DD>"
  [LAG_bus] -> Bus Selector8/1
  [NEWT_bus] -> Bus Selector9/1
  Bus Selector9/1 -> Mux5/2  "<y_DD>"
  Bus Selector10/1 -> Mux6/1  "<z_DD>"
  Bus Selector11/1 -> Mux6/2  "<z_DD>"
  [LAG_bus] -> Bus Selector10/1
  [NEWT_bus] -> Bus Selector11/1
  Bus Selector13/1 -> Mux7/2  "<phi_D>"
  [LAG_bus] -> Bus Selector12/1
  Bus Selector12/1 -> Mux7/1  "<phi_D>"
  [NEWT_bus] -> Bus Selector13/1
  Bus Selector14/1 -> Mux8/1  "<theta_D>"
  [NEWT_bus] -> Bus Selector15/1
  [LAG_bus] -> Bus Selector14/1
  Bus Selector15/1 -> Mux8/2  "<theta_D>"
  [NEWT_bus] -> Bus Selector17/1
  [LAG_bus] -> Bus Selector16/1
  Bus Selector17/1 -> Mux9/2  "<psi_D>"
  Bus Selector16/1 -> Mux9/1  "<psi_D>"
  Bus Selector19/1 -> Mux10/2  "<x_D>"
  [LAG_bus] -> Bus Selector18/1
  Bus Selector18/1 -> Mux10/1  "<x_D>"
  [NEWT_bus] -> Bus Selector19/1
  Bus Selector20/1 -> Mux11/1  "<y_D>"
  [LAG_bus] -> Bus Selector20/1
  [NEWT_bus] -> Bus Selector21/1
  Bus Selector21/1 -> Mux11/2  "<y_D>"
  [NEWT_bus] -> Bus Selector23/1
  Bus Selector23/1 -> Mux12/2  "<z_D>"
  [LAG_bus] -> Bus Selector22/1
  Bus Selector22/1 -> Mux12/1  "<z_D>"
  [NEWT_bus] -> Bus Selector25/1
  [LAG_bus] -> Bus Selector24/1
  Bus Selector24/1 -> Mux13/1  "<phi>"
  Bus Selector25/1 -> Mux13/2  "<phi>"
  [LAG_bus] -> Bus Selector26/1
  [NEWT_bus] -> Bus Selector27/1
  Bus Selector27/1 -> Mux14/2  "<theta>"
  Bus Selector26/1 -> Mux14/1  "<theta>"
  Bus Selector29/1 -> Mux15/2  "<psi>"
  Bus Selector28/1 -> Mux15/1  "<psi>"
  [LAG_bus] -> Bus Selector28/1
  [NEWT_bus] -> Bus Selector29/1
  Bus Selector31/1 -> Mux16/2  "<x>"
  Bus Selector30/1 -> Mux16/1  "<x>"
  [LAG_bus] -> Bus Selector30/1
  [NEWT_bus] -> Bus Selector31/1
  [NEWT_bus] -> Bus Selector33/1
  [LAG_bus] -> Bus Selector32/1
  Bus Selector32/1 -> Mux17/1  "<y>"
  Bus Selector33/1 -> Mux17/2  "<y>"
  [NEWT_bus] -> Bus Selector35/1
  Bus Selector35/1 -> Mux18/2  "<z>"
  [LAG_bus] -> Bus Selector34/1
  Bus Selector34/1 -> Mux18/1  "<z>"

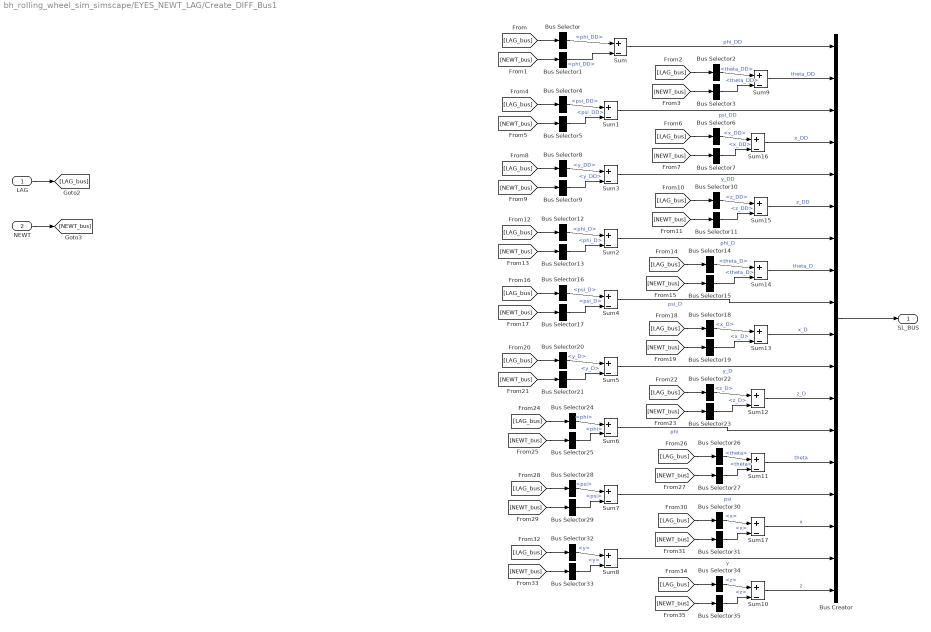
== system bh_rolling_wheel_sim_simscape/EYES_NEWT_LAG/Create_DIFF_Bus1 ==
  LAG : Inport
  NEWT : Inport  Port=2
  Bus Creator : BusCreator  Inputs=18
  Bus Selector : BusSelector  OutputSignals=phi_DD
  Bus Selector1 : BusSelector  OutputSignals=phi_DD
  Bus Selector10 : BusSelector  OutputSignals=z_DD
  Bus Selector11 : BusSelector  OutputSignals=z_DD
  Bus Selector12 : BusSelector  OutputSignals=phi_D
  Bus Selector13 : BusSelector  OutputSignals=phi_D
  Bus Selector14 : BusSelector  OutputSignals=theta_D
  Bus Selector15 : BusSelector  OutputSignals=theta_D
  Bus Selector16 : BusSelector  OutputSignals=psi_D
  Bus Selector17 : BusSelector  OutputSignals=psi_D
  Bus Selector18 : BusSelector  OutputSignals=x_D
  Bus Selector19 : BusSelector  OutputSignals=x_D
  Bus Selector2 : BusSelector  OutputSignals=theta_DD
  Bus Selector20 : BusSelector  OutputSignals=y_D
  Bus Selector21 : BusSelector  OutputSignals=y_D
  Bus Selector22 : BusSelector  OutputSignals=z_D
  Bus Selector23 : BusSelector  OutputSignals=z_D
  Bus Selector24 : BusSelector  OutputSignals=phi
  Bus Selector25 : BusSelector  OutputSignals=phi
  Bus Selector26 : BusSelector  OutputSignals=theta
  Bus Selector27 : BusSelector  OutputSignals=theta
  Bus Selector28 : BusSelector  OutputSignals=psi
  Bus Selector29 : BusSelector  OutputSignals=psi
  Bus Selector3 : BusSelector  OutputSignals=theta_DD
  Bus Selector30 : BusSelector  OutputSignals=x
  Bus Selector31 : BusSelector  OutputSignals=x
  Bus Selector32 : BusSelector  OutputSignals=y
  Bus Selector33 : BusSelector  OutputSignals=y
  Bus Selector34 : BusSelector  OutputSignals=z
  Bus Selector35 : BusSelector  OutputSignals=z
  Bus Selector4 : BusSelector  OutputSignals=psi_DD
  Bus Selector5 : BusSelector  OutputSignals=psi_DD
  Bus Selector6 : BusSelector  OutputSignals=x_DD
  Bus Selector7 : BusSelector  OutputSignals=x_DD
  Bus Selector8 : BusSelector  OutputSignals=y_DD
  Bus Selector9 : BusSelector  OutputSignals=y_DD
  Sum{,1..17} (18 alike) : Sum  Inputs=+|-
  SL_BUS : Outport
  wires:
  NEWT/1 -> [NEWT_bus]
  LAG/1 -> [LAG_bus]
  [LAG_bus] -> Bus Selector/1
  [NEWT_bus] -> Bus Selector1/1
  Bus Selector/1 -> Sum/1  "<phi_DD>"
  Bus Selector1/1 -> Sum/2  "<phi_DD>"
  Sum9/1 -> Bus Creator/2  "theta_DD"
  Sum6/1 -> Bus Creator/13  "phi"
  Sum10/1 -> Bus Creator/18  "z"
  Sum17/1 -> Bus Creator/16  "x"
  Sum7/1 -> Bus Creator/15  "psi"
  Sum4/1 -> Bus Creator/9  "psi_D"
  Sum14/1 -> Bus Creator/8  "theta_D"
  Sum12/1 -> Bus Creator/12  "z_D"
  Sum5/1 -> Bus Creator/11  "y_D"
  Sum8/1 -> Bus Creator/17  "y"
  Sum3/1 -> Bus Creator/5  "y_DD"
  Sum11/1 -> Bus Creator/14  "theta"
  Bus Creator/1 -> SL_BUS/1
  Sum2/1 -> Bus Creator/7  "phi_D"
  Sum13/1 -> Bus Creator/10  "x_D"
  Sum15/1 -> Bus Creator/6  "z_DD"
  Sum16/1 -> Bus Creator/4  "x_DD"
  Sum1/1 -> Bus Creator/3  "psi_DD"
  Sum/1 -> Bus Creator/1  "phi_DD"
  [LAG_bus] -> Bus Selector2/1
  [NEWT_bus] -> Bus Selector3/1
  Bus Selector2/1 -> Sum9/1  "<theta_DD>"
  Bus Selector3/1 -> Sum9/2  "<theta_DD>"
  [LAG_bus] -> Bus Selector4/1
  [NEWT_bus] -> Bus Selector5/1
  [NEWT_bus] -> Bus Selector7/1
  [LAG_bus] -> Bus Selector6/1
  [LAG_bus] -> Bus Selector8/1
  [NEWT_bus] -> Bus Selector9/1
  [LAG_bus] -> Bus Selector10/1
  [NEWT_bus] -> Bus Selector11/1
  [LAG_bus] -> Bus Selector12/1
  [NEWT_bus] -> Bus Selector13/1
  [NEWT_bus] -> Bus Selector15/1
  [LAG_bus] -> Bus Selector14/1
  [NEWT_bus] -> Bus Selector17/1
  [LAG_bus] -> Bus Selector16/1
  [LAG_bus] -> Bus Selector18/1
  [NEWT_bus] -> Bus Selector19/1
  [LAG_bus] -> Bus Selector20/1
  [NEWT_bus] -> Bus Selector21/1
  [NEWT_bus] -> Bus Selector23/1
  [LAG_bus] -> Bus Selector22/1
  [NEWT_bus] -> Bus Selector25/1
  [LAG_bus] -> Bus Selector24/1
  [LAG_bus] -> Bus Selector26/1
  [NEWT_bus] -> Bus Selector27/1
  [LAG_bus] -> Bus Selector28/1
  [NEWT_bus] -> Bus Selector29/1
  [LAG_bus] -> Bus Selector30/1
  [NEWT_bus] -> Bus Selector31/1
  [NEWT_bus] -> Bus Selector33/1
  [LAG_bus] -> Bus Selector32/1
  [NEWT_bus] -> Bus Selector35/1
  [LAG_bus] -> Bus Selector34/1
  Bus Selector4/1 -> Sum1/1  "<psi_DD>"
  Bus Selector5/1 -> Sum1/2  "<psi_DD>"
  Bus Selector8/1 -> Sum3/1  "<y_DD>"
  Bus Selector9/1 -> Sum3/2  "<y_DD>"
  Bus Selector12/1 -> Sum2/1  "<phi_D>"
  Bus Selector13/1 -> Sum2/2  "<phi_D>"
  Bus Selector16/1 -> Sum4/1  "<psi_D>"
  Bus Selector17/1 -> Sum4/2  "<psi_D>"
  Bus Selector20/1 -> Sum5/1  "<y_D>"
  Bus Selector21/1 -> Sum5/2  "<y_D>"
  Bus Selector24/1 -> Sum6/1  "<phi>"
  Bus Selector25/1 -> Sum6/2  "<phi>"
  Bus Selector28/1 -> Sum7/1  "<psi>"
  Bus Selector29/1 -> Sum7/2  "<psi>"
  Bus Selector32/1 -> Sum8/1  "<y>"
  Bus Selector33/1 -> Sum8/2  "<y>"
  Bus Selector6/1 -> Sum16/1  "<x_DD>"
  Bus Selector7/1 -> Sum16/2  "<x_DD>"
  Bus Selector10/1 -> Sum15/1  "<z_DD>"
  Bus Selector11/1 -> Sum15/2  "<z_DD>"
  Bus Selector14/1 -> Sum14/1  "<theta_D>"
  Bus Selector15/1 -> Sum14/2  "<theta_D>"
  Bus Selector18/1 -> Sum13/1  "<x_D>"
  Bus Selector19/1 -> Sum13/2  "<x_D>"
  Bus Selector22/1 -> Sum12/1  "<z_D>"
  Bus Selector23/1 -> Sum12/2  "<z_D>"
  Bus Selector26/1 -> Sum11/1  "<theta>"
  Bus Selector27/1 -> Sum11/2  "<theta>"
  Bus Selector30/1 -> Sum17/1  "<x>"
  Bus Selector31/1 -> Sum17/2  "<x>"
  Bus Selector34/1 -> Sum10/1  "<z>"
  Bus Selector35/1 -> Sum10/2  "<z>"

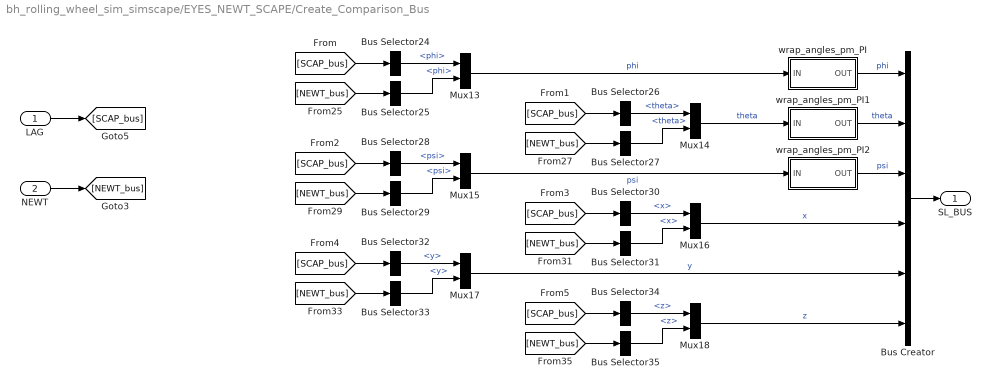
== system bh_rolling_wheel_sim_simscape/EYES_NEWT_SCAPE/Create_Comparison_Bus ==
  LAG : Inport
  NEWT : Inport  Port=2
  Bus Creator : BusCreator  Inputs=6
  Bus Selector24 : BusSelector  OutputSignals=phi
  Bus Selector25 : BusSelector  OutputSignals=phi
  Bus Selector26 : BusSelector  OutputSignals=theta
  Bus Selector27 : BusSelector  OutputSignals=theta
  Bus Selector28 : BusSelector  OutputSignals=psi
  Bus Selector29 : BusSelector  OutputSignals=psi
  Bus Selector30 : BusSelector  OutputSignals=x
  Bus Selector31 : BusSelector  OutputSignals=x
  Bus Selector32 : BusSelector  OutputSignals=y
  Bus Selector33 : BusSelector  OutputSignals=y
  Bus Selector34 : BusSelector  OutputSignals=z
  Bus Selector35 : BusSelector  OutputSignals=z
  Mux{13..18} (6 alike) : Mux  Inputs=2
  wrap_angles_pm_PI : Subsystem
  wrap_angles_pm_PI1 : Subsystem
  wrap_angles_pm_PI2 : Subsystem
  SL_BUS : Outport
  wires:
  NEWT/1 -> [NEWT_bus]
  LAG/1 -> [SCAP_bus]
  wrap_angles_pm_PI/1(OUT) -> Bus Creator/1  "phi"
  Mux18/1 -> Bus Creator/6  "z"
  Mux16/1 -> Bus Creator/4  "x"
  wrap_angles_pm_PI2/1(OUT) -> Bus Creator/3  "psi"
  Mux17/1 -> Bus Creator/5  "y"
  wrap_angles_pm_PI1/1(OUT) -> Bus Creator/2  "theta"
  Bus Creator/1 -> SL_BUS/1
  [NEWT_bus] -> Bus Selector25/1
  [SCAP_bus] -> Bus Selector24/1
  Bus Selector24/1 -> Mux13/1  "<phi>"
  Bus Selector25/1 -> Mux13/2  "<phi>"
  [SCAP_bus] -> Bus Selector26/1
  [NEWT_bus] -> Bus Selector27/1
  Bus Selector27/1 -> Mux14/2  "<theta>"
  Bus Selector26/1 -> Mux14/1  "<theta>"
  Bus Selector29/1 -> Mux15/2  "<psi>"
  Bus Selector28/1 -> Mux15/1  "<psi>"
  [SCAP_bus] -> Bus Selector28/1
  [NEWT_bus] -> Bus Selector29/1
  Bus Selector31/1 -> Mux16/2  "<x>"
  Bus Selector30/1 -> Mux16/1  "<x>"
  [SCAP_bus] -> Bus Selector30/1
  [NEWT_bus] -> Bus Selector31/1
  [NEWT_bus] -> Bus Selector33/1
  [SCAP_bus] -> Bus Selector32/1
  Bus Selector32/1 -> Mux17/1  "<y>"
  Bus Selector33/1 -> Mux17/2  "<y>"
  [NEWT_bus] -> Bus Selector35/1
  Bus Selector35/1 -> Mux18/2  "<z>"
  [SCAP_bus] -> Bus Selector34/1
  Bus Selector34/1 -> Mux18/1  "<z>"
  Mux15/1 -> wrap_angles_pm_PI2/1(IN)  "psi"
  Mux14/1 -> wrap_angles_pm_PI1/1(IN)  "theta"
  Mux13/1 -> wrap_angles_pm_PI/1(IN)  "phi"

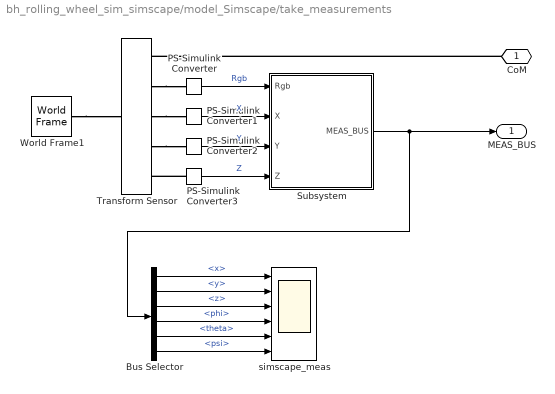
== system bh_rolling_wheel_sim_simscape/model_Simscape/take_measurements ==
  Bus Selector : BusSelector  OutputSignals=x,y,z,phi,theta,psi
  PS-Simulink Converter : nesl_utility/PS-Simulink Converter  PhysicalDomain=network_engine_domain  SubClassName=ps_output  LeftPortType=input  RightPortType=output  PseudoPeriodic=off  Frequencies=[]  VectorFormat=1-D array  Unit=m  AffineConversion=off
  PS-Simulink Converter1 : nesl_utility/PS-Simulink Converter  PhysicalDomain=network_engine_domain  SubClassName=ps_output  LeftPortType=input  RightPortType=output  PseudoPeriodic=off  Frequencies=[]  VectorFormat=1-D array  Unit=m  AffineConversion=off
  PS-Simulink Converter2 : nesl_utility/PS-Simulink Converter  PhysicalDomain=network_engine_domain  SubClassName=ps_output  LeftPortType=input  RightPortType=output  PseudoPeriodic=off  Frequencies=[]  VectorFormat=1-D array  Unit=m  AffineConversion=off
  PS-Simulink Converter3 : nesl_utility/PS-Simulink Converter  PhysicalDomain=network_engine_domain  SubClassName=ps_output  LeftPortType=input  RightPortType=output  PseudoPeriodic=off  Frequencies=[]  VectorFormat=1-D array  Unit=1  AffineConversion=off
  Subsystem : Subsystem
  Transform Sensor : sm_lib/Frames and Transforms/Transform Sensor  MeasurementFrame=World  SenseAngle=off  SenseAxis=off  SenseQ=off  SenseR=on  SenseRotationSequence=off  RotationSequence=XYX  SenseOmegaX=off  SenseOmegaY=off  SenseOmegaZ=off  SenseQDot=off  SenseRDot=off  SenseAlphaX=off  SenseAlphaY=off  SenseAlphaZ=off  SenseQDDot=off  SenseRDDot=off  SenseX=on  SenseY=on  SenseZ=on  SenseRad=off  SenseAzim=off  SenseDist=off  SenseInc=off  SenseXDot=off  SenseYDot=off  SenseZDot=off  SenseRadDot=off  SenseAzimDot=off  SenseDistDot=off  SenseIncDot=off  SenseXDDot=off  SenseYDDot=off  SenseZDDot=off  SenseRadDDot=off  SenseAzimDDot=off  SenseDistDDot=off  SenseIncDDot=off
  World Frame1 : sm_lib/Frames and Transforms/World Frame
  simscape_meas : Scope  NumInputPorts=6
  CoM : PMIOPort  Side=Right
  MEAS_BUS : Outport
  wires:
  Subsystem/1(MEAS_BUS) -> Bus Selector/1, MEAS_BUS/1
  Bus Selector/1 -> simscape_meas/1  "<x>"
  Bus Selector/2 -> simscape_meas/2  "<y>"
  Bus Selector/3 -> simscape_meas/3  "<z>"
  Bus Selector/4 -> simscape_meas/4  "<phi>"
  Bus Selector/5 -> simscape_meas/5  "<theta>"
  Bus Selector/6 -> simscape_meas/6  "<psi>"
  PS-Simulink Converter/1 -> Subsystem/1(Rgb)  "Rgb"
  PS-Simulink Converter1/1 -> Subsystem/2(X)  "X"
  PS-Simulink Converter2/1 -> Subsystem/3(Y)  "Y"
  PS-Simulink Converter3/1 -> Subsystem/4(Z)  "Z"
  connections:
  PS-Simulink Converter3/LConn1 -- Transform Sensor/RConn5
  Transform Sensor/RConn4 -- PS-Simulink Converter2/LConn1
  Transform Sensor/RConn2 -- PS-Simulink Converter/LConn1
  Transform Sensor/RConn3 -- PS-Simulink Converter1/LConn1
  World Frame1/RConn1 -- Transform Sensor/LConn1
  CoM/RConn1 -- Transform Sensor/RConn1

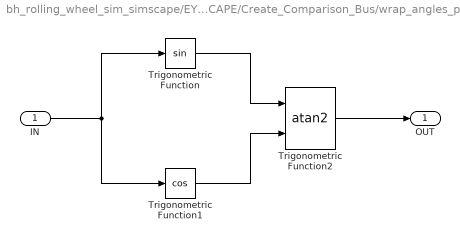
== system bh_rolling_wheel_sim_simscape/EYES_NEWT_SCAPE/Create_Comparison_Bus/wrap_angles_pm_PI ==
  IN : Inport
  Trigonometric Function : Trigonometry
  Trigonometric Function1 : Trigonometry  Operator=cos
  Trigonometric Function2 : Trigonometry  Operator=atan2
  OUT : Outport
  wires:
  IN/1 -> Trigonometric Function/1, Trigonometric Function1/1
  Trigonometric Function/1 -> Trigonometric Function2/1
  Trigonometric Function1/1 -> Trigonometric Function2/2
  Trigonometric Function2/1 -> OUT/1

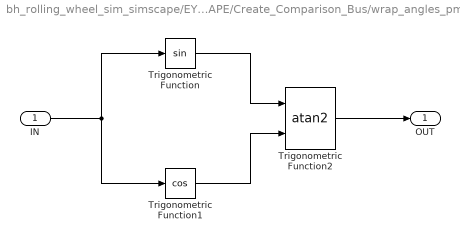
== system bh_rolling_wheel_sim_simscape/EYES_NEWT_SCAPE/Create_Comparison_Bus/wrap_angles_pm_PI1 ==
  IN : Inport
  Trigonometric Function : Trigonometry
  Trigonometric Function1 : Trigonometry  Operator=cos
  Trigonometric Function2 : Trigonometry  Operator=atan2
  OUT : Outport
  wires:
  IN/1 -> Trigonometric Function/1, Trigonometric Function1/1
  Trigonometric Function/1 -> Trigonometric Function2/1
  Trigonometric Function1/1 -> Trigonometric Function2/2
  Trigonometric Function2/1 -> OUT/1

== system bh_rolling_wheel_sim_simscape/EYES_NEWT_SCAPE/Create_Comparison_Bus/wrap_angles_pm_PI2 ==
  IN : Inport
  Trigonometric Function : Trigonometry
  Trigonometric Function1 : Trigonometry  Operator=cos
  Trigonometric Function2 : Trigonometry  Operator=atan2
  OUT : Outport
  wires:
  IN/1 -> Trigonometric Function/1, Trigonometric Function1/1
  Trigonometric Function/1 -> Trigonometric Function2/1
  Trigonometric Function1/1 -> Trigonometric Function2/2
  Trigonometric Function2/1 -> OUT/1

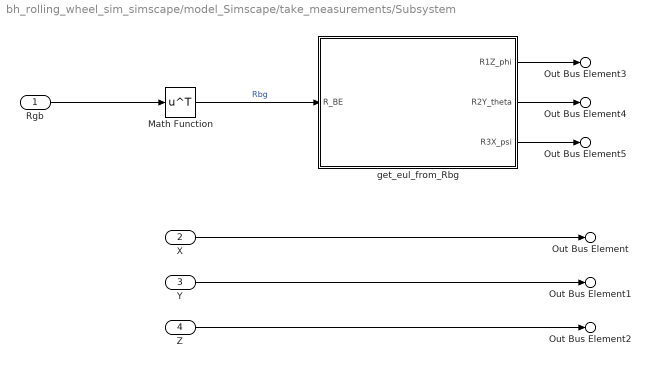
== system bh_rolling_wheel_sim_simscape/model_Simscape/take_measurements/Subsystem ==
  Rgb : Inport
  X : Inport  Port=2
  Y : Inport  Port=3
  Z : Inport  Port=4
  Math Function : Math  Operator=transpose
  get_eul_from_Rbg : MATLAB Function  TreatAsAtomicUnit=on
  Out Bus Element : Outport  PortName=MEAS_BUS  Element=x
  Out Bus Element1 : Outport  PortName=MEAS_BUS  Element=y
  Out Bus Element2 : Outport  PortName=MEAS_BUS  Element=z
  Out Bus Element3 : Outport  PortName=MEAS_BUS  Element=phi
  Out Bus Element4 : Outport  PortName=MEAS_BUS  Element=theta
  Out Bus Element5 : Outport  PortName=MEAS_BUS  Element=psi
  wires:
  Rgb/1 -> Math Function/1
  X/1 -> Out Bus Element/1
  Y/1 -> Out Bus Element1/1
  Z/1 -> Out Bus Element2/1
  get_eul_from_Rbg/3(R3X_psi) -> Out Bus Element5/1
  get_eul_from_Rbg/2(R2Y_theta) -> Out Bus Element4/1
  get_eul_from_Rbg/1(R1Z_phi) -> Out Bus Element3/1
  Math Function/1 -> get_eul_from_Rbg/1(R_BE)  "Rbg"

== matlab function bh_rolling_wheel_sim_simscape/model_Simscape/take_measurements/Subsystem/get_eul_from_Rbg ==
  data: R_BE input size=[3,3]; R1Z_phi output; R2Y_theta output; R3X_psi output
function [R1Z_phi, R2Y_theta, R3X_psi] = get_eul_from_RBE( R_BE )

   [R1Z_phi, R2Y_theta, R3X_psi] = bh_func_extract_euler_from_R_BE( R_BE );

end
